simulink model "lab2sm1"  (R2016a)
settings: Solver=VariableStepAuto  StartTime=0.0  StopTime=300  RelTol=1e-3
settings Model: Creator=Григорий  LastModifiedBy=Григорий

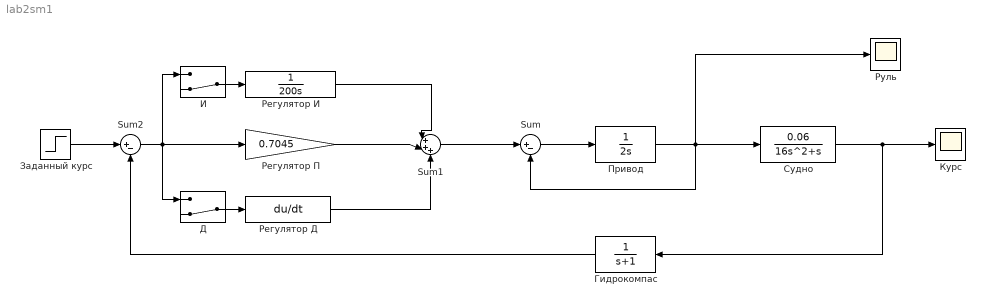
== system lab2sm1 ==
  Sum : Sum  Inputs=|+-
  Sum1 : Sum  Inputs=|+++
  Sum2 : Sum  Inputs=|+-
  "Гидрокомпас " : TransferFcn  Denominator=[1 1]
  Д : ManualSwitch  CurrentSetting=0
  Заданный курс : Step  Time=0  After=10  SampleTime=0
  И : ManualSwitch  CurrentSetting=0
  Курс : Scope
  Привод : TransferFcn  Denominator=[2 0]
  Регулятор Д : Derivative
  Регулятор И : TransferFcn  Denominator=[200 0]
  Регулятор П : Gain  Gain=0.7045
  Руль : Scope
  Судно : TransferFcn  Numerator=[0.06]  Denominator=[16 1 0]
  wires:
  Sum/1 -> Привод/1
  Sum1/1 -> Sum/1
  Привод/1 -> Sum/2, Руль/1, Судно/1
  Регулятор П/1 -> Sum1/2
  Sum2/1 -> И/1, Д/1, Регулятор П/1
  "Гидрокомпас "/1 -> Sum2/2
  Регулятор И/1 -> Sum1/1
  Регулятор Д/1 -> Sum1/3
  Д/1 -> Регулятор Д/1
  И/1 -> Регулятор И/1
  Заданный курс/1 -> Sum2/1
  Судно/1 -> "Гидрокомпас "/1, Курс/1
